simulink model "vipcodec"  (R2015b)
settings: Solver=FixedStepDiscrete  StartTime=0.0  StopTime=inf  RelTol=1e-3
values from neighbouring files (symbols this model uses):
  sz = size(I)    [TextDetectionExample.m]    (also in videopatternmatching.m = get(0,'ScreenSize'); videostabilize.m = fileInfo.VideoSize)
undefined symbols (not defined in the file or in its folder): gray, M, N
libraries: vipmisc x12, visionutilities x3, visionsinks x3, visiontransforms x2, visionanalysis x1, visionconversions x1, visionsources x1
settings Model: FPTRunName=Active  ExtModeAutoUpdateStatusClock=off  Creator=The MathWorks, Inc.  LastModifiedBy=The MathWorks, Inc.
settings DataIOCC: SaveFormat=Array  SaveOutput=off  SaveTime=off  SignalLoggingName=logsOut
settings OptimizationCC: DefaultParameterBehavior=Inlined  InlineInvariantSignals=on  ExpressionDepthLimit=2147483647  InitFltsAndDblsToZero=on  EfficientMapNaN2IntZero=off  BufferReusableBoundary=off
settings DebuggingCC: SaveWithParameterizedLinksMsg=none  UnderspecifiedInitializationDetection=Classic  MergeDetectMultiDrivingBlocksExec=none  CheckExecutionContextPreStartOutputMsg=on  CheckExecutionContextRuntimeOutputMsg=on  SignalResolutionControl=TryResolveAllWithWarning  MultiTaskDSMMsg=warning  MultiTaskCondExecSysMsg=none  FcnCallInpInsideContextMsg=UseLocalSettings  BusObjectLabelMismatch=none  StateNameClashWarn=warning  StrictBusMsg=None
settings HardwareCC: ProdBitPerPointer=32  ProdLargestAtomicFloat=None  ProdIntDivRoundTo=Undefined  ProdEndianess=Unspecified  ProdWordSize=32  ProdHWDeviceType=32-bit Generic  TargetBitPerLong=64  TargetBitPerPointer=64  TargetLongLongMode=on  TargetIntDivRoundTo=Zero  TargetEndianess=LittleEndian  TargetWordSize=64  TargetHWDeviceType=Generic->MATLAB Host Computer  ProdEqTarget=off
settings ModelReferenceCC: UpdateModelReferenceTargets=IfOutOfDate
settings SFSimCC: SimParseCustomCode=off
settings GRTTargetCC: TargetFcnLib=ansi_tfl_tmw.mat  GeneratePreprocessorConditionals=Disable all  CombineOutputUpdateFcns=off  GRTInterface=on
settings ConfigComp: CovMetricSettings=d  CovModelRefEnable=Off

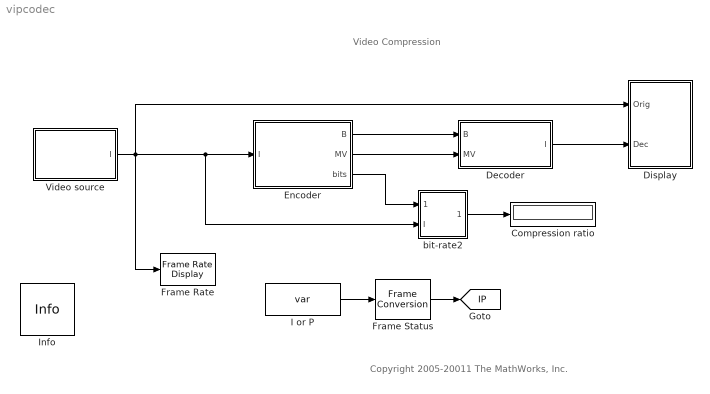
== system vipcodec ==
  note: Video Compression
  note: Copyright 2005-20011 The MathWorks, Inc.
  Compression ratio : Display
  Decoder : Subsystem
  Display : Subsystem
  Encoder : Subsystem
  Frame Rate : visionsinks/Frame Rate Display  UpdateRate=10
  Frame Status : FrameConversion  InheritSamplingMode=off  OutFrame=Sample-based
  I or P : FromWorkspace  VariableName=var  SampleTime=1/30  Interpolate=off  OutputAfterFinalValue=Cyclic repetition  mask{x=logical([0 0 1])}
      mask prompts: x "value"
      mask init:
      | dispVal=get_param(gcbh,'x');
      | var.time=[];
      | var.signals.values(1,1,1) = x(1);
      | var.signals.values(1,1,2) = x(2);
      | var.signals.values(1,1,3) = x(3);
      | var.signals.dimensions = [1 1];
      mask Display: disp(dispVal);
  Info : vipmisc/Info  SystemSampleTime=-1
  Video source : Subsystem
  bit-rate2 : Subsystem
  tag scope: IP=global
  wires:
  Encoder/1(B) -> Decoder/1(B)
  Encoder/2(MV) -> Decoder/2(MV)
  Video source/1(I) -> Encoder/1(I), bit-rate2/2(I), Display/1(Orig), Frame Rate/1
  Decoder/1(I) -> Display/2(Dec)
  Encoder/3(bits) -> bit-rate2/1(bits)
  bit-rate2/1(ratio) -> Compression ratio/1
  I or P/1 -> Frame Status/1
  Frame Status/1 -> [IP]

== system vipcodec/Decoder ==
  B : Inport
  MV : Inport  Port=2
  Block Processing : Subsystem  DialogController=vipDDGCreate  TreatAsAtomicUnit=on  mask(Block Processing){NumI=3, ParamPort=on, NumO=1, Blocksize={[15 1],[46 46],[1 2]}, Overlapsize={[0 0],[30 30],[0 0]}, Traverse=Row-wise}
      mask prompts: NumI "Number of inputs:"; ParamPort "Add port to supply subsystem parameters"; NumO "Number of outputs:"; Blocksize "Block size:"; Overlapsize "Overlap size:"; Traverse "Order of traversing:"
      mask help:
      | Repeats a user-specified operation on submatrices of the input matrix.
      |
      | This block extracts submatrices of a user-specified size from the input matrix. It sends each submatrix to a subsystem for processing, and then reassembles each subsystem output into the output matrix.
      |
      | Use the Block size and Overlap parameters to specify the size and overlap of each submatrix in cell array format.
      mask init:
      | errmsg = vipblkblockproc(gcbh, NumI, NumO, Blocksize, Overlapsize, Traverse, ParamPort);
      | error(errmsg);
      settings: CopyFcn=set_param(gcb,'LinkStatus','none');
      mask Help: eval('helpview(fullfile(docroot,''toolbox'',''vision'',''vision.map''),''vipblockprocessing'')');
      mask TypeOptions Traverse: Row-wise | Column-wise
      mask Display:
      | disp('Block\n Processing');
      | 
      | if ((NumI == 1) && ParamPort)
      |     port_label('input', 1, 'I');
      | end
      | 
      | if (NumI > 1)
      |     for (i = 1:NumI)
      |         port_label('input', i, ['I' int2str(i)]);
      |     end
      | end
      | 
      | if (ParamPort)
      |     port_label('input', NumI+1, 'P');
      | end
  Delay and pad : Subsystem
  I : Outport
  wires:
  B/1 -> Block Processing/1(In)
  Delay and pad/1(Out1) -> Block Processing/2(In2)
  MV/1 -> Block Processing/3(In3)
  Block Processing/1(Out) -> Delay and pad/1(In1), I/1
  [IP] -> Block Processing/4(P)

== system vipcodec/Display ==
  Orig : Inport
  Dec : Inport  Port=2
  Decoded : visionsinks/Video Viewer  inputType=Obsolete7b  imagePorts=One multidimensional signal  useColorMap=off  colormapValue=gray(256)  specRange=off  minInputVal=0  maxInputVal=255  FigPos=[769 490 160 136]  AxisZoom=on  trueSizedOnce=off  OpenAtMdlStart=on  DefaultConfigurationName=vipscopes.VideoViewerScopeCfg
  Original : visionsinks/Video Viewer  inputType=Obsolete7b  imagePorts=One multidimensional signal  useColorMap=off  colormapValue=gray(256)  specRange=off  minInputVal=0  maxInputVal=255  FigPos=[766 274 160 136]  AxisZoom=on  trueSizedOnce=off  OpenAtMdlStart=on  DefaultConfigurationName=vipscopes.VideoViewerScopeCfg
  wires:
  Orig/1 -> Original/1
  Dec/1 -> Decoded/1

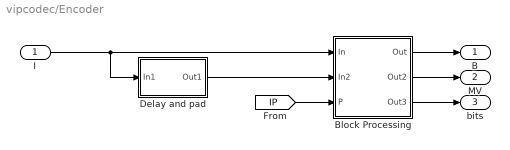
== system vipcodec/Encoder ==
  I : Inport
  Block Processing : Subsystem  DialogController=vipDDGCreate  TreatAsAtomicUnit=on  mask(Block Processing){NumI=2, ParamPort=on, NumO=3, Blocksize={[16 16],[46 46]}, Overlapsize={[0 0],[30 30]}, Traverse=Row-wise}
      mask prompts: NumI "Number of inputs:"; ParamPort "Add port to supply subsystem parameters"; NumO "Number of outputs:"; Blocksize "Block size:"; Overlapsize "Overlap size:"; Traverse "Order of traversing:"
      mask help:
      | Repeats a user-specified operation on submatrices of the input matrix.
      |
      | This block extracts submatrices of a user-specified size from the input matrix. It sends each submatrix to a subsystem for processing, and then reassembles each subsystem output into the output matrix.
      |
      | Use the Block size and Overlap parameters to specify the size and overlap of each submatrix in cell array format.
      mask init:
      | errmsg = vipblkblockproc(gcbh, NumI, NumO, Blocksize, Overlapsize, Traverse, ParamPort);
      | error(errmsg);
      settings: CopyFcn=set_param(gcb,'LinkStatus','none');
      mask Help: eval('helpview(fullfile(docroot,''toolbox'',''vision'',''vision.map''),''vipblockprocessing'')');
      mask TypeOptions Traverse: Row-wise | Column-wise
      mask Display:
      | disp('Block\n Processing');
      | 
      | if ((NumI == 1) && ParamPort)
      |     port_label('input', 1, 'I');
      | end
      | 
      | if (NumI > 1)
      |     for (i = 1:NumI)
      |         port_label('input', i, ['I' int2str(i)]);
      |     end
      | end
      | 
      | if (ParamPort)
      |     port_label('input', NumI+1, 'P');
      | end
  Delay and pad : Subsystem
  B : Outport
  MV : Outport  Port=2
  bits : Outport  Port=3
  wires:
  I/1 -> Delay and pad/1(In1), Block Processing/1(In)
  Block Processing/1(Out) -> B/1
  Delay and pad/1(Out1) -> Block Processing/2(In2)
  Block Processing/2(Out2) -> MV/1
  Block Processing/3(Out3) -> bits/1
  [IP] -> Block Processing/3(P)

== system vipcodec/Video source ==
  Image Data Type Conversion1 : visionconversions/Image Data Type Conversion  outDT=single  isSigned=on  wordLen=16  numFracBits=0
  Read Binary File : visionsources/Read Binary File  FileName=vipmen.bin  loopOrNot=on  numLoops=inf  VideoFormat=Custom  FOURCC=I420  BitStreamFormat=Planar  NumOutputs=3  ComponentOrder=[1 2 3]  Interlaced=off  LineOrdering=Top line first  Ts=1/30  Component1=Y'  Component2=Cb  Component3=Cr  Component4=Alpha  Bits1=8  Bits2=8  Bits3=8  Bits4=8  Rows1=120  Rows2=60  Rows3=60  Rows4=288  Cols1=160  Cols2=80  Cols3=80  Cols4=352  YRows=288  YCols=352  SignedOutput=off  FileEndian=Little endian  OutputEOF=off
  Selector2 : Selector  NumberOfDimensions=2  IndexMode=Zero-based  InputPortWidth=3  IndexOptions=Starting index (dialog),Starting index (dialog)  Indices=0,0  OutputSizes=112,160
  Terminator : Terminator
  Terminator1 : Terminator
  I : Outport
  wires:
  Image Data Type Conversion1/1 -> Selector2/1
  Selector2/1 -> I/1
  Read Binary File/1 -> Image Data Type Conversion1/1
  Read Binary File/2 -> Terminator/1
  Read Binary File/3 -> Terminator1/1

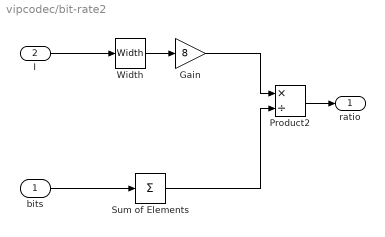
== system vipcodec/bit-rate2 ==
  bits : Inport
  I : Inport  Port=2
  Gain : Gain  Gain=8
  Product2 : Product  Inputs=*/  RndMeth=Zero
  Sum of Elements : Sum  Inputs=+  CollapseDim=2
  Width : Width
  ratio : Outport
  wires:
  Product2/1 -> ratio/1
  I/1 -> Width/1
  bits/1 -> Sum of Elements/1
  Sum of Elements/1 -> Product2/2
  Width/1 -> Gain/1
  Gain/1 -> Product2/1

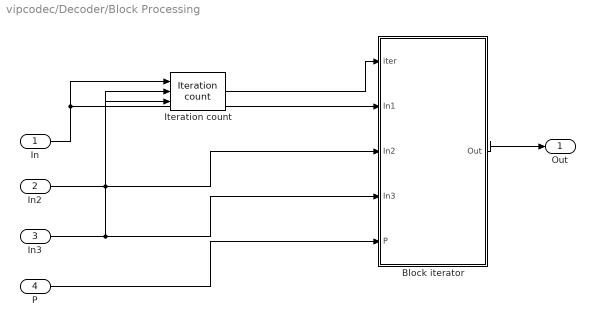
== system vipcodec/Decoder/Block Processing ==
  In : Inport
  In2 : Inport  Port=2
  In3 : Inport  Port=3
  P : Inport  Port=4
  Block iterator : Subsystem
      settings: CopyFcn=set_param(gcb,'ReferenceBlock','');
  Iteration count : vipmisc/Iteration count  NumI=NumI  blksize=Blocksize  ovlpsize=Overlapsize
  Out : Outport
  wires:
  Iteration count/1 -> Block iterator/1(iter)
  In/1 -> Iteration count/1, Block iterator/2(In1)
  Block iterator/1(Out) -> Out/1
  In2/1 -> Block iterator/3(In2), Iteration count/2
  In3/1 -> Block iterator/4(In3), Iteration count/3
  P/1 -> Block iterator/5(P)

== system vipcodec/Decoder/Delay and pad ==
  In1 : Inport
  2-D Pad : visionutilities/Image Pad  method=Constant  valSrc=Specify via dialog  value=0  spec=Pad size  rowDirection=Both left and right  outRowsMode=User-specified  rowSize=15  outColSize=10  colDirection=Both top and bottom  outColsMode=User-specified  colSize=15  outRowSize=12  trunc_flag=None
  Unit Delay : UnitDelay  SampleTime=-1
  Out1 : Outport
  wires:
  Unit Delay/1 -> 2-D Pad/1
  In1/1 -> Unit Delay/1
  2-D Pad/1 -> Out1/1

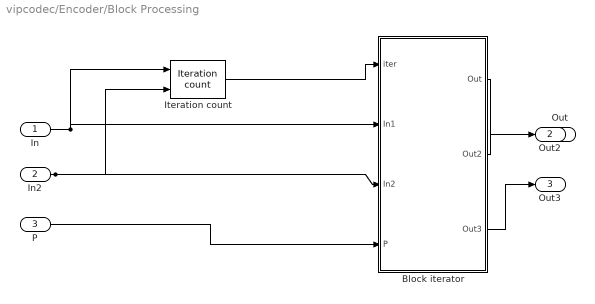
== system vipcodec/Encoder/Block Processing ==
  In : Inport
  In2 : Inport  Port=2
  P : Inport  Port=3
  Block iterator : Subsystem
      settings: CopyFcn=set_param(gcb,'ReferenceBlock','');
  Iteration count : vipmisc/Iteration count  NumI=NumI  blksize=Blocksize  ovlpsize=Overlapsize
  Out : Outport
  Out2 : Outport  Port=2
  Out3 : Outport  Port=3
  wires:
  P/1 -> Block iterator/4(P)
  Block iterator/3(Out3) -> Out3/1
  Block iterator/2(Out2) -> Out2/1
  In2/1 -> Iteration count/2, Block iterator/3(In2)
  Block iterator/1(Out) -> Out/1
  In/1 -> Block iterator/2(In1), Iteration count/1
  Iteration count/1 -> Block iterator/1(iter)

== system vipcodec/Encoder/Delay and pad ==
  In1 : Inport
  2-D Pad : visionutilities/Image Pad  method=Constant  valSrc=Specify via dialog  value=0  spec=Pad size  rowDirection=Both left and right  outRowsMode=User-specified  rowSize=15  outColSize=10  colDirection=Both top and bottom  outColsMode=User-specified  colSize=15  outRowSize=12  trunc_flag=None
  Unit Delay : UnitDelay  SampleTime=-1
  Out1 : Outport
  wires:
  In1/1 -> Unit Delay/1
  Unit Delay/1 -> 2-D Pad/1
  2-D Pad/1 -> Out1/1

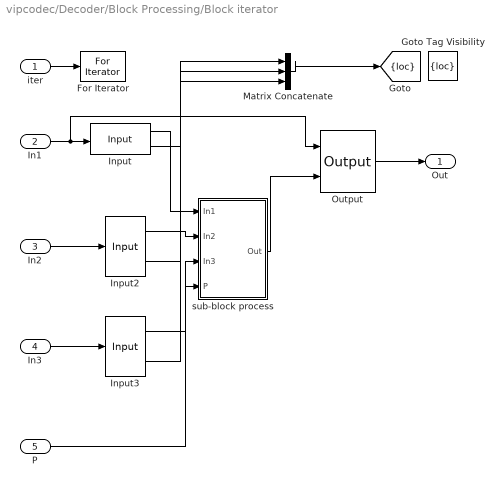
== system vipcodec/Decoder/Block Processing/Block iterator ==
  iter : Inport
  In1 : Inport  Port=2
  In2 : Inport  Port=3
  In3 : Inport  Port=4
  P : Inport  Port=5
  For Iterator : ForIterator  IterationSource=external  IterationLimit=(sz(1)/M)*(sz(2)/N)  ShowIterationPort=off  IndexMode=Zero-based  IterationVariableDataType=double
  Goto Tag Visibility : GotoTagVisibility  GotoTag=loc
  Input : vipmisc/Input  Blocksize=Blocksize{1}  Overlapsize=Overlapsize{1}  tverse=Row-wise
  Input2 : vipmisc/Input  Blocksize=Blocksize{2}  Overlapsize=Overlapsize{2}  tverse=Row-wise
  Input3 : vipmisc/Input  Blocksize=Blocksize{3}  Overlapsize=Overlapsize{3}  tverse=Row-wise
  Matrix Concatenate : Concatenate  NumInputs=3  Mode=Multidimensional array  ConcatenateDimension=2
  Output : vipmisc/Output  Blocksize=Blocksize{1}  Overlapsize=Overlapsize{1}  tverse=Row-wise
  sub-block process : Subsystem
  Out : Outport
  tag scope: loc=scoped
  wires:
  Matrix Concatenate/1 -> [loc]
  Input/2 -> Matrix Concatenate/1
  Input/1 -> sub-block process/1(In1)
  iter/1 -> For Iterator/1
  In1/1 -> Input/1, Output/1
  Output/1 -> Out/1
  sub-block process/1(Out) -> Output/2
  Input2/2 -> Matrix Concatenate/2
  In2/1 -> Input2/1
  Input2/1 -> sub-block process/2(In2)
  Input3/2 -> Matrix Concatenate/3
  In3/1 -> Input3/1
  Input3/1 -> sub-block process/3(In3)
  P/1 -> sub-block process/4(P)

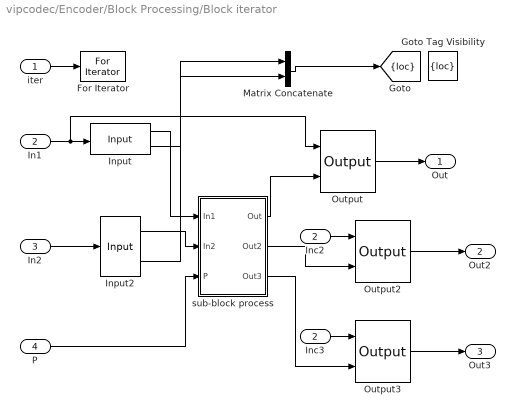
== system vipcodec/Encoder/Block Processing/Block iterator ==
  iter : Inport
  In1 : Inport  Port=2
  In2 : Inport  Port=3
  P : Inport  Port=4
  For Iterator : ForIterator  IterationSource=external  IterationLimit=(sz(1)/M)*(sz(2)/N)  ShowIterationPort=off  IndexMode=Zero-based  IterationVariableDataType=double
  Goto Tag Visibility : GotoTagVisibility  GotoTag=loc
  Inc2 : InportShadow  Port=2
  Inc3 : InportShadow  Port=2
  Input : vipmisc/Input  Blocksize=Blocksize{1}  Overlapsize=Overlapsize{1}  tverse=Row-wise
  Input2 : vipmisc/Input  Blocksize=Blocksize{2}  Overlapsize=Overlapsize{2}  tverse=Row-wise
  Matrix Concatenate : Concatenate  Mode=Multidimensional array  ConcatenateDimension=2
  Output : vipmisc/Output  Blocksize=Blocksize{1}  Overlapsize=Overlapsize{1}  tverse=Row-wise
  Output2 : vipmisc/Output  Blocksize=Blocksize{1}  Overlapsize=Overlapsize{1}  tverse=Row-wise
  Output3 : vipmisc/Output  Blocksize=Blocksize{1}  Overlapsize=Overlapsize{1}  tverse=Row-wise
  sub-block process : Subsystem
  Out : Outport
  Out2 : Outport  Port=2
  Out3 : Outport  Port=3
  tag scope: loc=scoped
  wires:
  P/1 -> sub-block process/3(P)
  sub-block process/3(Out3) -> Output3/2
  Output3/1 -> Out3/1
  Inc3/1 -> Output3/1
  sub-block process/2(Out2) -> Output2/2
  Output2/1 -> Out2/1
  Inc2/1 -> Output2/1
  Input2/1 -> sub-block process/2(In2)
  In2/1 -> Input2/1
  Input2/2 -> Matrix Concatenate/2
  sub-block process/1(Out) -> Output/2
  Output/1 -> Out/1
  In1/1 -> Output/1, Input/1
  iter/1 -> For Iterator/1
  Input/1 -> sub-block process/1(In1)
  Input/2 -> Matrix Concatenate/1
  Matrix Concatenate/1 -> [loc]

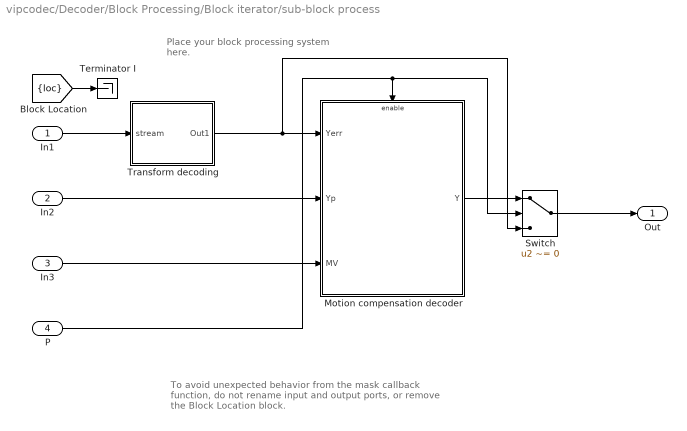
== system vipcodec/Decoder/Block Processing/Block iterator/sub-block process ==
  note: To avoid unexpected behavior from the mask
      | callback function, do not rename input and output ports,
      | or remove the Block Location block.
  note: Place your block
      | processing system here.
  In1 : Inport
  In2 : Inport  Port=2
  In3 : Inport  Port=3
  P : Inport  Port=4
  Motion compensation decoder : Subsystem
  Switch : Switch  Criteria=u2 ~= 0
  Terminator I : Terminator
  Transform decoding : Subsystem
  Out : Outport
  wires:
  [loc] -> Terminator I/1
  In1/1 -> Transform decoding/1(stream)
  Transform decoding/1(Out1) -> Switch/3, Motion compensation decoder/1(Yerr)
  In2/1 -> Motion compensation decoder/2(Yp)
  In3/1 -> Motion compensation decoder/3(MV)
  P/1 -> Motion compensation decoder/Enable, Switch/2
  Motion compensation decoder/1(Y) -> Switch/1
  Switch/1 -> Out/1

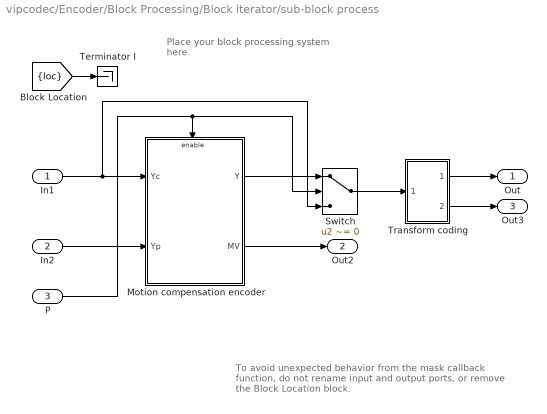
== system vipcodec/Encoder/Block Processing/Block iterator/sub-block process ==
  note: Place your block
      | processing system here.
  note: To avoid unexpected behavior from the mask
      | callback function, do not rename input and output ports,
      | or remove the Block Location block.
  In1 : Inport
  In2 : Inport  Port=2
  P : Inport  Port=3
  Motion compensation encoder : Subsystem
  Switch : Switch  Criteria=u2 ~= 0
  Terminator I : Terminator
  Transform coding : Subsystem
  Out : Outport
  Out2 : Outport  Port=2
  Out3 : Outport  Port=3
  wires:
  [loc] -> Terminator I/1
  P/1 -> Switch/2, Motion compensation encoder/Enable
  In1/1 -> Switch/3, Motion compensation encoder/1(Yc)
  In2/1 -> Motion compensation encoder/2(Yp)
  Motion compensation encoder/1(Y) -> Switch/1
  Motion compensation encoder/2(MV) -> Out2/1
  Switch/1 -> Transform coding/1(In1)
  Transform coding/1(stream) -> Out/1
  Transform coding/2(bits) -> Out3/1

== system vipcodec/Decoder/Block Processing/Block iterator/sub-block process/Motion compensation decoder ==
  Yerr : Inport
  Yp : Inport  Port=2
  MV : Inport  Port=3
  Enable : EnablePort  PropagateVarSize=During execution
  SelectMatch3 : Subsystem
  Sum5 : Sum  Inputs=|++
  Y : Outport
  wires:
  MV/1 -> SelectMatch3/2(Indx)
  Yp/1 -> SelectMatch3/1(Image)
  Sum5/1 -> Y/1
  SelectMatch3/1(Out) -> Sum5/1
  Yerr/1 -> Sum5/2

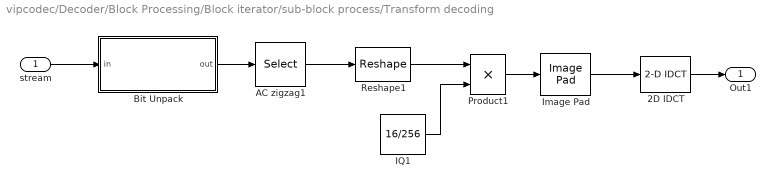
== system vipcodec/Decoder/Block Processing/Block iterator/sub-block process/Transform decoding ==
  stream : Inport
  2D IDCT : visiontransforms/2-D IDCT  CompMethod=Table lookup  Dimension=0  TableOpt=Speed  BitRevOrder=off  SkipNorm=off  firstCoeffDataTypeStr=Inherit: Same word length as input  firstCoeffLastDataTypeStr=Inherit: Same word length as input  outputMin=[]  outputMax=[]  roundingMode=Floor  overflowMode=off
  AC zigzag1 : Selector  IndexOptions=Index vector (dialog)  Indices="[1     3     4    10    11    21    22    36     2     5     9    12    20    23    35    37     6     8    13    19    24    34    38    49     7    14    18    25    33    39    48    50    15    17    26    32    40    47    51     58    16    27    31    41    46    52    57    59    28    30    42    45     53    56    60    63    29    43    44    54    55    61    62    64]"  OutputSizes=1
  Bit Unpack : MATLAB Function  TreatAsAtomicUnit=on
  IQ1 : Constant  Value=16/256  VectorParams1D=off  OutDataTypeStr=Inherit: Inherit via back propagation
  Image Pad : visionutilities/Image Pad  method=Constant  valSrc=Specify via dialog  value=0  spec=Pad size  rowDirection=Right  outRowsMode=User-specified  rowSize=8  outColSize=10  colDirection=Bottom  outColsMode=User-specified  colSize=8  outRowSize=12  trunc_flag=None
  Product1 : Product  SaturateOnIntegerOverflow=on  RndMeth=Zero  OutDataTypeStr=Inherit: Same as first input
  Reshape1 : Reshape  OutputDimensionality=Customize  OutputDimensions=[8,8]
  Out1 : Outport
  wires:
  AC zigzag1/1 -> Reshape1/1
  Bit Unpack/1(out) -> AC zigzag1/1
  2D IDCT/1 -> Out1/1
  stream/1 -> Bit Unpack/1(in)
  Image Pad/1 -> 2D IDCT/1
  Reshape1/1 -> Product1/1
  Product1/1 -> Image Pad/1
  IQ1/1 -> Product1/2

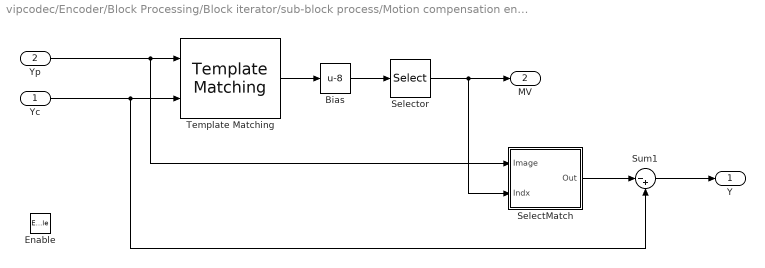
== system vipcodec/Encoder/Block Processing/Block iterator/sub-block process/Motion compensation encoder ==
  Yc : Inport
  Yp : Inport  Port=2
  Enable : EnablePort  PropagateVarSize=During execution
  Bias : Bias  Bias=-8
  SelectMatch : Subsystem
  Selector : Selector  InputPortWidth=2  IndexOptions=Index vector (dialog)  Indices=[2 1]  OutputSizes=1
  Sum1 : Sum  Inputs=|-+  OutDataTypeStr=Inherit: Same as first input
  Template Matching : visionanalysis/Template Matching  metric=Sum of absolute differences  output=Best match location  method=Three-step  nMetric=off  nSize=3  roi=off  roiValid=off  accumMode=Binary point scaling  accumWordLength=32  accumFracLength=0  prodOutputMode=Binary point scaling  prodOutputWordLength=32  prodOutputFracLength=0  roundingMode=Floor  overflowMode=off
  Y : Outport
  MV : Outport  Port=2
  wires:
  Sum1/1 -> Y/1
  SelectMatch/1(Out) -> Sum1/1
  Yc/1 -> Sum1/2, Template Matching/2
  Yp/1 -> SelectMatch/1(Image), Template Matching/1
  Template Matching/1 -> Bias/1
  Bias/1 -> Selector/1
  Selector/1 -> SelectMatch/2(Indx), MV/1

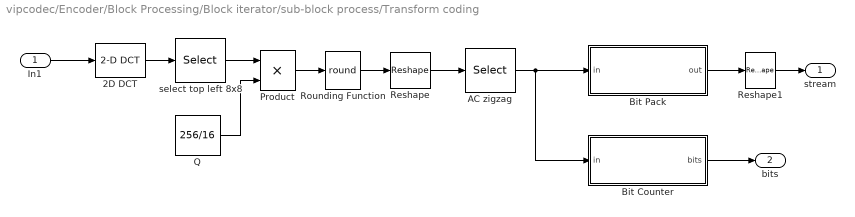
== system vipcodec/Encoder/Block Processing/Block iterator/sub-block process/Transform coding ==
  In1 : Inport
  2D DCT : visiontransforms/2-D DCT  CompMethod=Table lookup  Dimension=0  TableOpt=Speed  BitRevOrder=off  SkipNorm=off  firstCoeffDataTypeStr=Inherit: Same word length as input  firstCoeffLastDataTypeStr=Inherit: Same word length as input  outputMin=[]  outputMax=[]  roundingMode=Floor  overflowMode=off
  AC zigzag : Selector  IndexOptions=Index vector (dialog)  Indices="[0  8     1     2     9    16    24    17    10     3     4    11    18    25  32    40    33    26    19    12     5     6    13    20    27    34    41  48    56    49    42    35    28    21    14     7    15    22    29    36  43    50    57    58    51    44    37    30    23    31    38    45    52  59    60    53    46    39    47    54    61    62    55    63]+1"  OutputSizes=1
  Bit Counter : MATLAB Function  TreatAsAtomicUnit=on
  Bit Pack : MATLAB Function  TreatAsAtomicUnit=on
  Product : Product  SaturateOnIntegerOverflow=on  RndMeth=Zero  OutDataTypeStr=Inherit: Same as first input
  Q : Constant  Value=256/16  VectorParams1D=off  OutDataTypeStr=Inherit: Inherit via back propagation
  Reshape : Reshape  OutputDimensionality=Column vector (2-D)  OutputDimensions=[8,8]
  Reshape1 : Reshape  OutputDimensionality=Column vector (2-D)  OutputDimensions=[8,8]
  Rounding Function : Rounding  Operator=round
  select top left 8x8 : Selector  NumberOfDimensions=2  IndexMode=Zero-based  IndexOptions=Starting index (dialog),Starting index (dialog)  Indices=0,0  OutputSizes=8,8
  stream : Outport
  bits : Outport  Port=2
  wires:
  Reshape/1 -> AC zigzag/1
  Reshape1/1 -> stream/1
  2D DCT/1 -> select top left 8x8/1
  In1/1 -> 2D DCT/1
  AC zigzag/1 -> Bit Counter/1(in), Bit Pack/1(in)
  Product/1 -> Rounding Function/1
  Rounding Function/1 -> Reshape/1
  select top left 8x8/1 -> Product/1
  Bit Counter/1(bits) -> bits/1
  Q/1 -> Product/2
  Bit Pack/1(out) -> Reshape1/1

== system vipcodec/Decoder/Block Processing/Block iterator/sub-block process/Motion compensation decoder/SelectMatch3 ==
  Image : Inport
  Indx : Inport  Port=2
  Selector3 : Selector  NumberOfDimensions=2  IndexMode=Zero-based  InputPortWidth=3  IndexOptions=Starting index (port),Starting index (port)  Indices=1,1  OutputSizes=16,16
  Selector4 : Selector  InputPortWidth=2  IndexOptions=Index vector (dialog)  Indices=1  OutputSizes=1
  Selector5 : Selector  InputPortWidth=2  IndexOptions=Index vector (dialog)  Indices=2  OutputSizes=1
  Out : Outport
  wires:
  Selector4/1 -> Selector3/2
  Selector5/1 -> Selector3/3
  Image/1 -> Selector3/1
  Indx/1 -> Selector4/1, Selector5/1
  Selector3/1 -> Out/1

== system vipcodec/Encoder/Block Processing/Block iterator/sub-block process/Motion compensation encoder/SelectMatch ==
  Image : Inport
  Indx : Inport  Port=2
  Selector3 : Selector  NumberOfDimensions=2  IndexMode=Zero-based  InputPortWidth=3  IndexOptions=Starting index (port),Starting index (port)  Indices=1,1  OutputSizes=16,16
  Selector4 : Selector  InputPortWidth=2  IndexOptions=Index vector (dialog)  Indices=1  OutputSizes=1
  Selector5 : Selector  InputPortWidth=2  IndexOptions=Index vector (dialog)  Indices=2  OutputSizes=1
  Out : Outport
  wires:
  Selector3/1 -> Out/1
  Indx/1 -> Selector5/1, Selector4/1
  Image/1 -> Selector3/1
  Selector5/1 -> Selector3/3
  Selector4/1 -> Selector3/2

== matlab function vipcodec/Encoder/Block Processing/Block iterator/sub-block process/Transform coding/Bit Counter ==
  data: in input; bits output
function bits = bitcounter(in)
% This bitcounter assumes that the input signal will be 
% huffman encoded and counts bits based on this assumption. Note 
% however that the Bit Pack and Bit Unpack blocks only perform
% run length encoding.

numacbits = 0;
run = 0;

dclen = [2, 3, 3, 3, 3, 3, 4, 5, 6, 7, 8, 9];

if (in(1) < 0) 
    dcval = uint32(-in(1)); 
else
    dcval = uint32(in(1)); 
end

for i=0:11
    if (dcval == 0) 
        break; 
    end
    dcval = uint32(bitshift(dcval,-1));
end
numdcbits = dclen(i+1) + i;

aclen = [2,  2,  3,  4,  5,  7,  8, 10, 16, 16,...
    4,  5,  7,  9, 11, 16, 16, 16, 16, 16,...
    5,  8, 10, 12, 16, 16, 16, 16, 16, 16,...
    6,  9, 12, 16, 16, 16, 16, 16, 16, 16,...
    6, 10, 16, 16, 16, 16, 16, 16, 16, 16,...
    7, 11, 16, 16, 16, 16, 16, 16, 16, 16,...
    7, 12, 16, 16, 16, 16, 16, 16, 16, 16,...
    8, 12, 16, 16, 16, 16, 16, 16, 16, 16,...
    9, 15, 16, 16, 16, 16, 16, 16, 16, 16,...
    9, 16, 16, 16, 16, 16, 16, 16, 16, 16,...
    9, 16, 16, 16, 16, 16, 16, 16, 16, 16,...
    10, 16, 16, 16, 16, 16, 16, 16, 16, 16,...
    10, 16, 16, 16, 16, 16, 16, 16, 16, 16,...
    11, 16, 16, 16, 16, 16, 16, 16, 16, 16,...
    16, 16, 16, 16, 16, 16, 16, 16, 16, 16,...
    16, 16, 16, 16, 16, 16, 16, 16, 16, 16];



for i=1:63
    if (in(i+1) == 0)
        run = run+1;
        if (i < 63)
            continue;
        end
    end
    
    if (in(i+1) < 0) 
        acval = uint32(-in(i+1)); 
    else
        acval = uint32(in(i+1));
    end

    for j=0:31
        if (acval == 0) 
            break; 
        end

        acval = uint32(bitshift(acval,-1));
    end
    
    while (run > 15)
        run = run-15;
        numacbits = numacbits+11;
    end

    numacbits = numacbits + aclen(run*10 + j+1) + j;
    run = 0;
end

if (run > 0) 
    numacbits = numacbits+4; 
end
     
bits = single(numacbits+numdcbits);

== matlab function vipcodec/Encoder/Block Processing/Block iterator/sub-block process/Transform coding/Bit Pack ==
  data: in input; out output uint32 size=15
function out=bitpack(in) 

% Pack output bits into given length using run length coding. The first 
% coefficient (DC) is coded using 32 bits. The AC coefficients are run 
% length coded using 4 bits for run and 8 bits for value. The output is uint32.

persistent prev_out;
if isempty(prev_out)
    prev_out = uint32(zeros(15,1));
end
    out=uint32(prev_out);
    % Bit Pack Routine  
    bitpos=int32(0); 
    Temp= uint32(0); 
    run =  uint32(0); 
    outpos = 2; 
    pval=single(0); 
    cval=single(0);
  
    numcoefs = 64;
    
    out1 =  int32(fix(in(1)));
    
    if out1>=-1   
       out(1) = uint32(out1);
    else
       out(1) = uint32(intmax('uint32') - uint32(abs(out1)) +uint32(2));
    end

    % ac coefficients
    % 4 bit - run length followed by 8 bit coef value  
    pval(:) = fix(in(2)+0.5);
    if (pval > 127),  pval(:) = 127; end % saturate  
    if (pval < -128), pval(:) = -128; end

    run(:) = 0;
    for i=(3): numcoefs   
        cval(:) = floor(in(i)+0.5); 
        if (pval == cval && run < 14)  
            run(:)=run(:)+1;
        else  
            [flag, bitpos, out, Temp, outpos] = putbits(bitpos, out, Temp, outpos, run, 4);
            if (~flag) 
                prev_out=out;
                return; 
            end

            if (pval > 127),  pval(:) = 127;  end % saturate  
            if (pval < -128), pval(:) = -128; end
            pval(:) = pval+128; % make positive  

            [flag, bitpos, out, Temp, outpos] = putbits(bitpos, out, Temp, outpos, uint32(pval), 8);
            if (~flag) 
                prev_out=out;
                return; 
            end

            run(:) = 0;
        end
        pval(:) = cval;
    end

    % last coefficient  
    [flag, bitpos, out, Temp, outpos] = putbits(bitpos, out, Temp, outpos, run, 4);
    if (~flag) 
        prev_out=out;
        return; 
    end

    if (pval > 127),  pval(:) = 127;  end % saturate 
    if (pval < -128), pval(:) = -128; end
    pval(:) = pval+128; % make positive 

    [flag, bitpos, out, Temp, outpos] = putbits(bitpos, out, Temp, outpos, pval, 8);
    if (~flag) 
        prev_out=out;
        return; 
    end

    [bitpos, out, Temp, outpos] = flushbits(bitpos, out, Temp, outpos);%#ok
    prev_out=out;
end

%%========================================================================
function [flag, bitposO, outO, TempO, outposO] = putbits(bitpos, out, Temp, outpos, val, bits)
     
    valIn = uint32(val);
    bitsIn=int32(bits);
    bitposO = int32(bitpos);
    outO = uint32(out);
    TempO = uint32(Temp);
    outposO = outpos;
    
    if (bitposO + bitsIn > 32)  
        bitsleft = int32(32 - bitposO);
        bval=uint32(0);
        bval(:) = bitshift(valIn, -(bitsIn-bitsleft)); 
        TempO(:) = bitor(TempO,bval); 
        outO(outposO) = TempO;
        outposO = outposO+1;
        if (outposO > length(out))  
            flag = 0;
            return;
        end
        TempO = uint32(0);
        bitposO(:) = int32(0);
        bitsIn(:) = bitsIn-bitsleft; 
        valIn(:)=bitshift(valIn, 32-bitsIn);  
        valIn(:)=bitshift(valIn, -(32-bitsIn)); 
    end
    valIn(:)=bitshift(valIn, (32-(bitsIn+(bitposO))));  
    TempO = bitor(TempO, valIn); 
    bitposO(:) = bitposO + bitsIn;
    flag=1;
end

%%========================================================================
function [bitposO, outO, TempO, outposO, out] = flushbits(bitpos, out, Temp, outpos)
 
    [flag, bitposO, outO, TempO, outposO] = putbits(bitpos, out, Temp, outpos, 15, 4);
    if (~flag) 
        return; 
    end
    if (outposO > length(out)+1), return; end
    outO(outposO) = TempO;
end

== matlab function vipcodec/Decoder/Block Processing/Block iterator/sub-block process/Transform decoding/Bit Unpack ==
  data: in input; out output single size=64
function out=bitunpack(in)

% Unpack the bits packed by the bit pack block. If there are not enough 
% values in the packed stream the rest of the output is filled with zeros.

persistent prev_out;
if isempty(prev_out)
    prev_out = single(zeros(64,1));
end
    out = prev_out;
    cbits= int32(0); 
    inpos=2; 
    Temp = uint32(0); 
    run = uint32(0);
    val = uint32(0);
   
    numcoefs = 64;
    if bitget(in(1),32)%negative
        out(1)=-int32(intmax('uint32')- uint32(in(1))) - int32(1);
    else
        out(1)=int32(in(1));
    end
    
    % ac coefficients
    % 4 bit - run length followed by 8 bit coef value  
    i=2;
    while (i<=numcoefs)   
         
        [flag, cbits, inpos, Temp, run] = getbits(cbits, inpos, Temp, in, run, 4);
        if (~flag) 
            break; 
        end
        if (run == 15), break;   end % end of stream  
        
        [flag, cbits, inpos, Temp, val] = getbits(cbits, inpos, Temp, in, val, 8);
        if (~flag) 
            break; 
        end 
        
        for j= i: min(run+i, numcoefs)    
            out(j) = single(single(val)-128.0);  
        end
        i = i + double(run)+1;
    end

    % when we havent got all coefs in the stream 
    for j=i:numcoefs    
        out(i) = 0;
    end
    prev_out(:)=out;
end

%%=================================================
function [flag, cbitsO, inposO, TempO, valO] = getbits(cbits, inpos, Temp, in, val, bits)

    lval = uint32(0); 
    temp = uint32(0);
    cbitsO = int32(cbits);
    inposO = inpos;
    TempO = uint32(Temp);
    valO = uint32(val);
    inwidth = length(in);
    if (cbitsO < bits)  
        if (inposO > inwidth) 
            flag=0;
            return; 
        end

        lval(:) =  bitshift(TempO, -(32-cbitsO));  
        bits(:) = bits - cbitsO;
        TempO = in(inposO); inposO = inposO +1;  
        lval = bitshift(lval, bits);  
        cbitsO(:) = int32(32);
    end

    temp(:) = bitshift(TempO, -(32-bits));  
    TempO(:) = bitshift(TempO, bits);  
    valO(:) = bitor(lval, temp); 
    cbitsO(:) = cbitsO - bits;

    flag = 1;
end
